simulink model "regulator_pid"  (R2013a)
settings: Solver=ode45  StartTime=0.0  StopTime=10.0  MaxStep=0.01  RelTol=1e-3
values from neighbouring files (symbols this model uses):
  Kr = 4    [lab4.m]
  stan = 0    [lab4.m]
  tau = 0.7    [lab4.m]
  Td = 3    [lab4.m]    (also in skrypt.m = 5)
  Ti = 2    [lab4.m]
settings Model: Creator=L13-3  LastModifiedBy=Dawid Perdek
settings DataIOCC: SignalLoggingSaveFormat=ModelDataLogs
settings DebuggingCC: UnderspecifiedInitializationDetection=Simplified  MultiTaskDSMMsg=warning  MultiTaskCondExecSysMsg=none  StateNameClashWarn=none  StrictBusMsg=ErrorOnBusTreatedAsVector  NonBusSignalsTreatedAsBus=error
settings RTWCC: IncludeERTFirstTime=on
settings GRTTargetCC: CodeReplacementLibrary=None  CPPClassGenCompliant=on

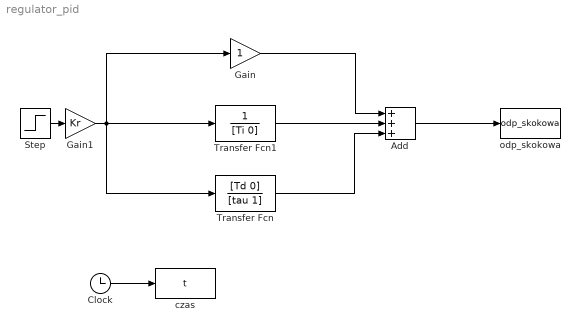
== system regulator_pid ==
  Add : Sum  Inputs=+++
  Clock : Clock
  Gain : Gain
  Gain1 : Gain  Gain=Kr
  Step : Step  Time=stan  SampleTime=0
  Transfer Fcn : TransferFcn  Numerator=[Td 0]  Denominator=[tau 1]
  Transfer Fcn1 : TransferFcn  Denominator=[Ti 0]
  czas : ToWorkspace  VariableName=t  SampleTime=-1
  odp_skokowa : ToWorkspace  VariableName=odp_skokowa  SampleTime=-1
  wires:
  Step/1 -> Gain1/1
  Gain/1 -> Add/1
  Add/1 -> odp_skokowa/1
  Clock/1 -> czas/1
  Transfer Fcn/1 -> Add/3
  Gain1/1 -> Transfer Fcn1/1, Transfer Fcn/1, Gain/1
  Transfer Fcn1/1 -> Add/2
